simulink model "l64_dev"  (Simulink 7.9)
settings: Solver=ode45  StartTime=0.0  StopTime=525000  RelTol=1e-3
undefined symbols (not defined in the file): sfp
libraries: xbsIndex_r4 x835, xps_library x23, casper_library_delays x22, casper_library_misc x3
(part 1 of 8)
settings Model: Creator=jkocz  LastModifiedBy=jkocz
settings DebuggingCC: FcnCallInpInsideContextMsg=Use local settings  StrictBusMsg=Warning
settings GRTTargetCC: CombineOutputUpdateFcns=off  GRTInterface=on

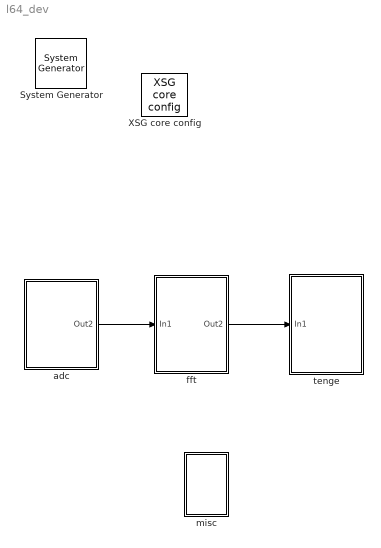
== system l64_dev ==
  " System Generator" : xbsIndex_r4/ System Generator  Tag=genX  xilinxfamily=virtex6  part=xc6vsx475t  speed=-1  package=ff1759  synthesis_tool=XST  clock_wrapper=Clock Enables  directory=./l64_dev/sysgen  proj_type=Project Navigator  Synth_file=XST Defaults  Impl_file=ISE Defaults  testbench=off  simulink_period=1  sysclk_period=5  dcm_input_clock_period=100  incr_netlist=off  trim_vbits=Everywhere in SubSystem  dbl_ovrd=According to Block Masks  core_generation=According to Block Masks  run_coregen=off  deprecated_control=off  eval_field=0  block_type=sysgen
      settings: block_version=11.4
  XSG core config : xps_library/XSG core config  Tag=xps:xsg  hw_sys=ROACH2:sx475t  clk_src=adc0_clk  ROACH_clk_src=adc0_clk  ROACH2_clk_src=adc0_clk  clk_rate=200  sample_period=1  synthesis_tool=XST
  adc : Subsystem
  fft : Subsystem
  misc : Subsystem
  tenge : Subsystem
  wires:
  adc/1(Out2) -> fft/1(In1)
  fft/1(Out2) -> tenge/1(In1)

== system l64_dev/adc ==
  Constant2 : Constant  Value=0
  Constant3 : Constant  Value=0
  Mux : Mux  Inputs=2
  Out2 : Outport
  wires:
  Mux/1 -> Out2/1
  Constant2/1 -> Mux/1
  Constant3/1 -> Mux/2

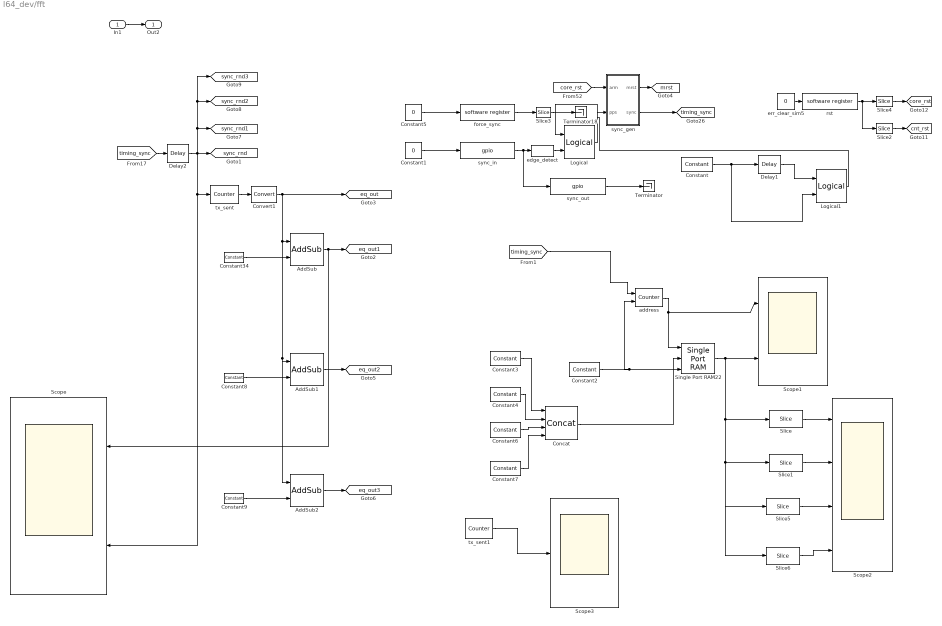
== system l64_dev/fft ==
  In1 : Inport
  AddSub : xbsIndex_r4/AddSub  mode=Addition  use_carryin=off  use_carryout=off  en=off  latency=0  precision=User Defined  arith_type=Unsigned  n_bits=64  bin_pt=0  quantization=Truncate  overflow=Wrap  dbl_ovrd=off  use_behavioral_HDL=off  hw_selection=Fabric  pipelined=off  block_type=addsub
  AddSub1 : xbsIndex_r4/AddSub  mode=Addition  use_carryin=off  use_carryout=off  en=off  latency=0  precision=User Defined  arith_type=Unsigned  n_bits=64  bin_pt=0  quantization=Truncate  overflow=Wrap  dbl_ovrd=off  use_behavioral_HDL=off  hw_selection=Fabric  pipelined=off  block_type=addsub
  AddSub2 : xbsIndex_r4/AddSub  mode=Addition  use_carryin=off  use_carryout=off  en=off  latency=0  precision=User Defined  arith_type=Unsigned  n_bits=64  bin_pt=0  quantization=Truncate  overflow=Wrap  dbl_ovrd=off  use_behavioral_HDL=off  hw_selection=Fabric  pipelined=off  block_type=addsub
  Concat : xbsIndex_r4/Concat  num_inputs=4  dbl_ovrd=off  block_type=concat
  Constant : xbsIndex_r4/Constant  const=1  gui_display_data_type=Boolean  arith_type=Boolean  n_bits=16  bin_pt=14  preci_type=Single  exp_width=8  frac_width=24  explicit_period=on  period=1  equ=P=C  opselect=C  inp2=PCIN>>17  opr=+  inp1=P  carry=CIN  dbl_ovrd=off  block_type=constant
  Constant1 : Constant  Value=0  SampleTime=1/4
  Constant2 : xbsIndex_r4/Constant  const=1  gui_display_data_type=Boolean  arith_type=Boolean  n_bits=16  bin_pt=14  preci_type=Single  exp_width=8  frac_width=24  explicit_period=on  period=1  equ=P=C  opselect=C  inp2=PCIN>>17  opr=+  inp1=P  carry=CIN  dbl_ovrd=off  block_type=constant
  Constant{3..4,6..7} (4 alike) : xbsIndex_r4/Constant  const=65536  gui_display_data_type=Fixed-point  arith_type=Unsigned  n_bits=16  bin_pt=0  preci_type=Single  exp_width=8  frac_width=24  explicit_period=on  period=1  equ=P=C  opselect=C  inp2=PCIN>>17  opr=+  inp1=P  carry=CIN  dbl_ovrd=off  block_type=constant
  Constant34 : xbsIndex_r4/Constant  const=8192  gui_display_data_type=Fixed-point  arith_type=Unsigned  n_bits=14  bin_pt=0  preci_type=Single  exp_width=8  frac_width=24  explicit_period=on  period=1  equ=P=C  opselect=C  inp2=PCIN>>17  opr=+  inp1=P  carry=CIN  dbl_ovrd=off  block_type=constant
  Constant5 : Constant  Value=0  SampleTime=1/4
  Constant8 : xbsIndex_r4/Constant  const=16384  gui_display_data_type=Fixed-point  arith_type=Unsigned  n_bits=15  bin_pt=0  preci_type=Single  exp_width=8  frac_width=24  explicit_period=on  period=1  equ=P=C  opselect=C  inp2=PCIN>>17  opr=+  inp1=P  carry=CIN  dbl_ovrd=off  block_type=constant
  Constant9 : xbsIndex_r4/Constant  const=24576  gui_display_data_type=Fixed-point  arith_type=Unsigned  n_bits=16  bin_pt=0  preci_type=Single  exp_width=8  frac_width=24  explicit_period=on  period=1  equ=P=C  opselect=C  inp2=PCIN>>17  opr=+  inp1=P  carry=CIN  dbl_ovrd=off  block_type=constant
  Convert1 : xbsIndex_r4/Convert  gui_display_data_type=Fixed-point  arith_type=Unsigned  n_bits=64  bin_pt=0  float_type=Single  exp_bits=8  fraction_bits=24  quantization=Truncate  overflow=Wrap  en=off  latency=0  dbl_ovrd=off  pipeline=off  block_type=convert
      settings: block_version=11.4
  Delay1 : xbsIndex_r4/Delay  rst=off  infoeditControl=Selection of Reset will increase slice count due to use of real FFs and instead of SRLs  en=off  latency=2  dbl_ovrd=off  reg_retiming=on  block_type=delay
  Delay2 : xbsIndex_r4/Delay  rst=off  infoeditControl=Selection of Reset will increase slice count due to use of real FFs and instead of SRLs  en=off  latency=10  dbl_ovrd=off  reg_retiming=on  block_type=delay
  Logical : xbsIndex_r4/Logical  logical_function=OR  inputs=2  en=off  latency=0  precision=Full  arith_type=Unsigned  n_bits=16  bin_pt=0  align_bp=on  dbl_ovrd=off  block_type=logical
  Logical1 : xbsIndex_r4/Logical  logical_function=OR  inputs=2  en=off  latency=0  precision=Full  arith_type=Unsigned  n_bits=16  bin_pt=0  align_bp=on  dbl_ovrd=off  block_type=logical
  Scope : Scope  NumInputPorts=2
      settings: YMin=0~-1  YMax=2e+19~1
  Scope1 : Scope  NumInputPorts=2
      settings: YMin=0~0  YMax=200~8500
  Scope2 : Scope  NumInputPorts=4
      settings: YMin=0~0~-5~-5  YMax=200~8500~5~5  SaveName=ScopeData2
  Scope3 : Scope
      settings: YMin=0  YMax=200  SaveName=ScopeData6
  Single Port RAM22 : xbsIndex_r4/Single Port RAM  depth=200  initVector=0  distributed_mem=Block RAM  write_mode=Read Before Write  rst=off  init_reg=0  en=off  latency=1  dbl_ovrd=off  optimize=Area  use_rpm=on  block_type=spram
  Slice : xbsIndex_r4/Slice  nbits=16  boolean_output=off  mode=Upper Bit Location + Width  bit1=0  base1=MSB of Input  bit0=0  base0=LSB of Input  dbl_ovrd=off  block_type=slice
  Slice1 : xbsIndex_r4/Slice  nbits=16  boolean_output=off  mode=Lower Bit Location + Width  bit1=0  base1=MSB of Input  bit0=32  base0=LSB of Input  dbl_ovrd=off  block_type=slice
  Slice2 : xbsIndex_r4/Slice  nbits=1  boolean_output=on  mode=Lower Bit Location + Width  bit1=0  base1=MSB of Input  bit0=0  base0=LSB of Input  dbl_ovrd=off  block_type=slice
      settings: block_version=10.1.3
  Slice3 : xbsIndex_r4/Slice  nbits=1  boolean_output=on  mode=Lower Bit Location + Width  bit1=0  base1=MSB of Input  bit0=0  base0=LSB of Input  dbl_ovrd=off  block_type=slice
      settings: block_version=10.1.3
  Slice4 : xbsIndex_r4/Slice  nbits=1  boolean_output=on  mode=Lower Bit Location + Width  bit1=0  base1=MSB of Input  bit0=1  base0=LSB of Input  dbl_ovrd=off  block_type=slice
      settings: block_version=10.1.3
  Slice5 : xbsIndex_r4/Slice  nbits=16  boolean_output=off  mode=Lower Bit Location + Width  bit1=0  base1=MSB of Input  bit0=16  base0=LSB of Input  dbl_ovrd=off  block_type=slice
  Slice6 : xbsIndex_r4/Slice  nbits=16  boolean_output=off  mode=Lower Bit Location + Width  bit1=0  base1=MSB of Input  bit0=0  base0=LSB of Input  dbl_ovrd=off  block_type=slice
  Terminator : Terminator
  Terminator18 : Terminator
  address : xbsIndex_r4/Counter  cnt_type=Count Limited  cnt_to=199  operation=Up  start_count=0  cnt_by_val=1  arith_type=Unsigned  n_bits=8  bin_pt=0  load_pin=off  rst=on  en=on  explicit_period=on  period=1  dbl_ovrd=off  use_behavioral_HDL=off  implementation=Fabric  block_type=counter
      settings: block_version=11.4
  edge_detect : casper_library_misc/edge_detect  edge=Rising  polarity=Active High  x_in=[0 0.08 0.08 0.16 0.16 0.24 0.24 0.32 0.32 0.4]  y_in="[-1 -1  1  1  1  1  1  1  1  1]"  x_out=[0.6 0.68 0.68 0.76 0.76 0.84 0.84 0.92 0.92 1]  y_out="[-1 -1  1  1 -1 -1 -1 -1 -1 -1]"
  err_clear_sim5 : Constant  Value=0
  force_sync : xps_library/software register  Tag=xps:sw_reg  io_dir=From Processor  arith_type=Unsigned  bitwidth=32  bin_pt=0  sample_period=1  gw_name=l64_dev_fft_force_sync_user_data_out
      link override r_10gbe_demo_gbe_core_rst_user_data_out: arith_type=Unsigned  n_bits=32  bin_pt=0  period=1
      link override r_10gbe_test_cnt_rst_user_data_out: arith_type=Unsigned  n_bits=32  bin_pt=0  period=1
      link override r_10gbe_test_gbe_core_rst_user_data_out: arith_type=Unsigned  n_bits=32  bin_pt=0  period=1
      link override r_xaui_test_cnt_rst_user_data_out: arith_type=Unsigned  n_bits=32  bin_pt=0  period=1
  rst : xps_library/software register  Tag=xps:sw_reg  io_dir=From Processor  arith_type=Unsigned  bitwidth=32  bin_pt=0  sample_period=1  gw_name=l64_dev_fft_rst_user_data_out
      link override r_10gbe_demo_gbe_core_rst_user_data_out: arith_type=Unsigned  n_bits=32  bin_pt=0  period=1
      link override r_10gbe_test_cnt_rst_user_data_out: arith_type=Unsigned  n_bits=32  bin_pt=0  period=1
      link override r_10gbe_test_gbe_core_rst_user_data_out: arith_type=Unsigned  n_bits=32  bin_pt=0  period=1
      link override r_xaui_test_cnt_rst_user_data_out: arith_type=Unsigned  n_bits=32  bin_pt=0  period=1
  sync_gen : Subsystem  mask(sync_gen_hw){sync_period_bits=14}
      mask prompts: sync_period_bits "Size of sync generator counter (bits)"
      mask help:
      | This circuit implements a scheme for synchronizing a design to within an FPGA clock of an external 1 pulse-per-second signal.
      |
      | * An arm pulse will cause the sync_gen to stop issuing sync pulses.
      | * It will then ignore the next input trigger (1PPS), while sync is flushed through the DSP pipeline.
      | * It will then lock onto the next trigger (1PPS) and issue syncs thereafter every sync_period clocks.
      | * You will need a multiple of (pfb_fir taps*LCM(FFT reorder orders) *fft bins/parallel inputs). See the sync memo for further details.
  sync_in : xps_library/gpio  Tag=xps:gpio  io_group=ROACH2:sync_in  io_dir=in  arith_type=Boolean  bitwidth=1  bin_pt=0  bit_index=0  sample_period=1  use_single_ended=off  use_ddr=off  reg_iob=on  reg_clk_phase=0  termination=None
  sync_out : xps_library/gpio  Tag=xps:gpio  io_group=ROACH2:sync_out  io_dir=out  arith_type=Boolean  bitwidth=1  bin_pt=0  bit_index=0  sample_period=1  use_single_ended=off  use_ddr=off  reg_iob=on  reg_clk_phase=0  termination=None
  tx_sent : xbsIndex_r4/Counter  cnt_type=Free Running  cnt_to=Inf  operation=Up  start_count=0  cnt_by_val=1  arith_type=Unsigned  n_bits=13  bin_pt=0  load_pin=off  rst=on  en=off  explicit_period=on  period=1  dbl_ovrd=off  use_behavioral_HDL=off  implementation=Fabric  block_type=counter
      settings: block_version=11.4
  tx_sent1 : xbsIndex_r4/Counter  cnt_type=Count Limited  cnt_to=10  operation=Up  start_count=0  cnt_by_val=1  arith_type=Unsigned  n_bits=13  bin_pt=0  load_pin=off  rst=off  en=off  explicit_period=on  period=1  dbl_ovrd=off  use_behavioral_HDL=off  implementation=Fabric  block_type=counter
      settings: block_version=11.4
  Out2 : Outport
  tag scope: cnt_rst=global, core_rst=global, eq_out1=global, eq_out2=global, eq_out3=global, eq_out=global, mrst=global, sync_rnd1=global, sync_rnd2=global, sync_rnd3=global, sync_rnd=global, timing_sync=global
  wires:
  In1/1 -> Out2/1
  [timing_sync] -> Delay2/1
  tx_sent/1 -> Convert1/1
  sync_gen/1(mrst) -> [mrst]
  sync_gen/2(sync) -> [timing_sync]
  [core_rst] -> sync_gen/1(arm)
  err_clear_sim5/1 -> rst/1
  rst/1 -> Slice4/1, Slice2/1
  Slice2/1 -> [cnt_rst]
  Slice4/1 -> [core_rst]
  force_sync/1 -> Slice3/1
  Constant5/1 -> force_sync/1
  Constant1/1 -> sync_in/1
  Logical/1 -> sync_gen/2(pps)
  sync_in/1 -> sync_out/1, edge_detect/1
  sync_out/1 -> Terminator/1
  edge_detect/1 -> Logical/2
  Slice3/1 -> Terminator18/1
  Constant/1 -> Delay1/1, Logical1/2
  Delay1/1 -> Logical1/1
  Logical1/1 -> Logical/1
  Delay2/1 -> [sync_rnd], tx_sent/1, Scope/2, [sync_rnd3], [sync_rnd2], [sync_rnd1]
  Constant2/1 -> Single Port RAM22/3, address/2
  Single Port RAM22/1 -> Scope1/2, Slice/1, Slice1/1, Slice5/1, Slice6/1
  address/1 -> Single Port RAM22/1, Scope1/1
  [timing_sync] -> address/1
  Convert1/1 -> [eq_out], AddSub/1, AddSub1/1, AddSub2/1
  Constant3/1 -> Concat/1
  Constant4/1 -> Concat/2
  Constant6/1 -> Concat/3
  Constant7/1 -> Concat/4
  Concat/1 -> Single Port RAM22/2
  Slice/1 -> Scope2/1
  Slice1/1 -> Scope2/2
  Slice5/1 -> Scope2/3
  Slice6/1 -> Scope2/4
  Constant34/1 -> AddSub/2
  AddSub/1 -> [eq_out1], Scope/1
  Constant8/1 -> AddSub1/2
  AddSub1/1 -> [eq_out2]
  Constant9/1 -> AddSub2/2
  AddSub2/1 -> [eq_out3]
  tx_sent1/1 -> Scope3/1

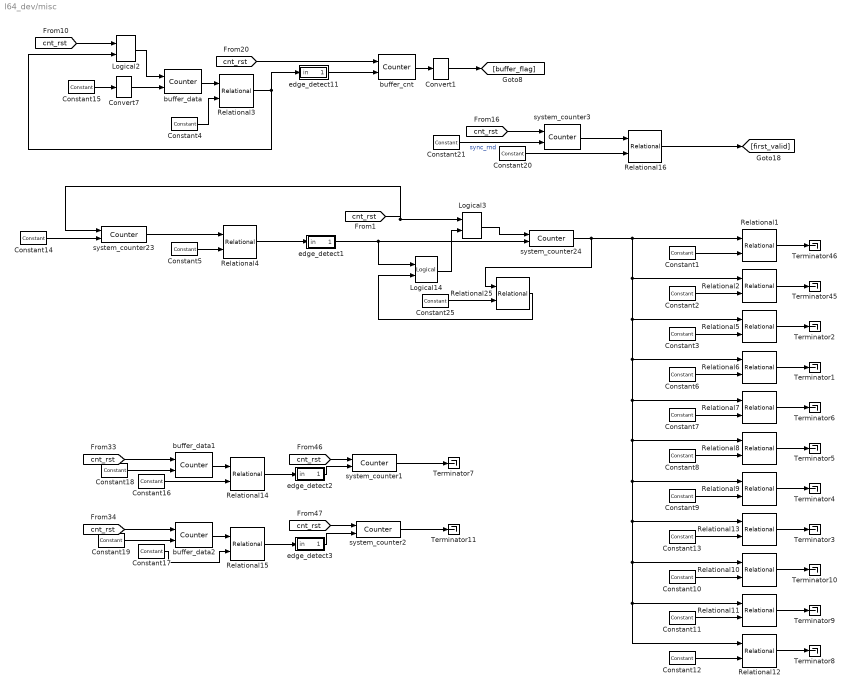
== system l64_dev/misc ==
  Constant1 : xbsIndex_r4/Constant  const=0  gui_display_data_type=Fixed-point  arith_type=Unsigned  n_bits=3  bin_pt=0  preci_type=Single  exp_width=8  frac_width=24  explicit_period=on  period=1  equ=P=C  opselect=C  inp2=PCIN>>17  opr=+  inp1=P  carry=CIN  dbl_ovrd=off  block_type=constant
  Constant10 : xbsIndex_r4/Constant  const=8  gui_display_data_type=Fixed-point  arith_type=Unsigned  n_bits=4  bin_pt=0  preci_type=Single  exp_width=8  frac_width=24  explicit_period=on  period=1  equ=P=C  opselect=C  inp2=PCIN>>17  opr=+  inp1=P  carry=CIN  dbl_ovrd=off  block_type=constant
  Constant11 : xbsIndex_r4/Constant  const=9  gui_display_data_type=Fixed-point  arith_type=Unsigned  n_bits=4  bin_pt=0  preci_type=Single  exp_width=8  frac_width=24  explicit_period=on  period=1  equ=P=C  opselect=C  inp2=PCIN>>17  opr=+  inp1=P  carry=CIN  dbl_ovrd=off  block_type=constant
  Constant{12,16..17,25} (4 alike) : xbsIndex_r4/Constant  const=10  gui_display_data_type=Fixed-point  arith_type=Unsigned  n_bits=4  bin_pt=0  preci_type=Single  exp_width=8  frac_width=24  explicit_period=on  period=1  equ=P=C  opselect=C  inp2=PCIN>>17  opr=+  inp1=P  carry=CIN  dbl_ovrd=off  block_type=constant
  Constant13 : xbsIndex_r4/Constant  const=7  gui_display_data_type=Fixed-point  arith_type=Unsigned  n_bits=3  bin_pt=0  preci_type=Single  exp_width=8  frac_width=24  explicit_period=on  period=1  equ=P=C  opselect=C  inp2=PCIN>>17  opr=+  inp1=P  carry=CIN  dbl_ovrd=off  block_type=constant
  Constant{14..15,18..19,21} (5 alike) : xbsIndex_r4/Constant  const=0  gui_display_data_type=Boolean  arith_type=Boolean  n_bits=9  bin_pt=0  preci_type=Single  exp_width=8  frac_width=24  explicit_period=on  period=1  equ=P=C  opselect=C  inp2=PCIN>>17  opr=+  inp1=P  carry=CIN  dbl_ovrd=off  block_type=constant
  Constant2 : xbsIndex_r4/Constant  const=1  gui_display_data_type=Fixed-point  arith_type=Unsigned  n_bits=3  bin_pt=0  preci_type=Single  exp_width=8  frac_width=24  explicit_period=on  period=1  equ=P=C  opselect=C  inp2=PCIN>>17  opr=+  inp1=P  carry=CIN  dbl_ovrd=off  block_type=constant
  Constant20 : xbsIndex_r4/Constant  const=1  gui_display_data_type=Fixed-point  arith_type=Unsigned  n_bits=2  bin_pt=0  preci_type=Single  exp_width=8  frac_width=24  explicit_period=on  period=1  equ=P=C  opselect=C  inp2=PCIN>>17  opr=+  inp1=P  carry=CIN  dbl_ovrd=off  block_type=constant
  Constant3 : xbsIndex_r4/Constant  const=2  gui_display_data_type=Fixed-point  arith_type=Unsigned  n_bits=3  bin_pt=0  preci_type=Single  exp_width=8  frac_width=24  explicit_period=on  period=1  equ=P=C  opselect=C  inp2=PCIN>>17  opr=+  inp1=P  carry=CIN  dbl_ovrd=off  block_type=constant
  Constant4 : xbsIndex_r4/Constant  const=22  gui_display_data_type=Fixed-point  arith_type=Unsigned  n_bits=5  bin_pt=0  preci_type=Single  exp_width=8  frac_width=24  explicit_period=on  period=1  equ=P=C  opselect=C  inp2=PCIN>>17  opr=+  inp1=P  carry=CIN  dbl_ovrd=off  block_type=constant
  Constant5 : xbsIndex_r4/Constant  const=109  gui_display_data_type=Fixed-point  arith_type=Unsigned  n_bits=9  bin_pt=0  preci_type=Single  exp_width=8  frac_width=24  explicit_period=on  period=1  equ=P=C  opselect=C  inp2=PCIN>>17  opr=+  inp1=P  carry=CIN  dbl_ovrd=off  block_type=constant
  Constant6 : xbsIndex_r4/Constant  const=3  gui_display_data_type=Fixed-point  arith_type=Unsigned  n_bits=3  bin_pt=0  preci_type=Single  exp_width=8  frac_width=24  explicit_period=on  period=1  equ=P=C  opselect=C  inp2=PCIN>>17  opr=+  inp1=P  carry=CIN  dbl_ovrd=off  block_type=constant
  Constant7 : xbsIndex_r4/Constant  const=4  gui_display_data_type=Fixed-point  arith_type=Unsigned  n_bits=3  bin_pt=0  preci_type=Single  exp_width=8  frac_width=24  explicit_period=on  period=1  equ=P=C  opselect=C  inp2=PCIN>>17  opr=+  inp1=P  carry=CIN  dbl_ovrd=off  block_type=constant
  Constant8 : xbsIndex_r4/Constant  const=5  gui_display_data_type=Fixed-point  arith_type=Unsigned  n_bits=3  bin_pt=0  preci_type=Single  exp_width=8  frac_width=24  explicit_period=on  period=1  equ=P=C  opselect=C  inp2=PCIN>>17  opr=+  inp1=P  carry=CIN  dbl_ovrd=off  block_type=constant
  Constant9 : xbsIndex_r4/Constant  const=6  gui_display_data_type=Fixed-point  arith_type=Unsigned  n_bits=3  bin_pt=0  preci_type=Single  exp_width=8  frac_width=24  explicit_period=on  period=1  equ=P=C  opselect=C  inp2=PCIN>>17  opr=+  inp1=P  carry=CIN  dbl_ovrd=off  block_type=constant
  Convert1 : xbsIndex_r4/Convert  gui_display_data_type=Boolean  arith_type=Boolean  n_bits=64  bin_pt=0  float_type=Single  exp_bits=8  fraction_bits=24  quantization=Truncate  overflow=Wrap  en=off  latency=0  dbl_ovrd=off  pipeline=off  block_type=convert
      settings: block_version=11.4
  Convert7 : xbsIndex_r4/Convert  gui_display_data_type=Boolean  arith_type=Boolean  n_bits=64  bin_pt=0  float_type=Single  exp_bits=8  fraction_bits=24  quantization=Truncate  overflow=Wrap  en=off  latency=0  dbl_ovrd=off  pipeline=off  block_type=convert
      settings: block_version=11.4
  Logical14 : xbsIndex_r4/Logical  logical_function=AND  inputs=2  en=off  latency=0  precision=Full  arith_type=Unsigned  n_bits=16  bin_pt=0  align_bp=on  dbl_ovrd=off  block_type=logical
      settings: block_version=11.4
  Logical2 : xbsIndex_r4/Logical  logical_function=OR  inputs=2  en=off  latency=1  precision=Full  arith_type=Unsigned  n_bits=16  bin_pt=0  align_bp=on  dbl_ovrd=off  block_type=logical
      settings: block_version=11.4
  Logical3 : xbsIndex_r4/Logical  logical_function=OR  inputs=2  en=off  latency=1  precision=Full  arith_type=Unsigned  n_bits=16  bin_pt=0  align_bp=on  dbl_ovrd=off  block_type=logical
      settings: block_version=11.4
  Relational{1..15,25} (16 alike) : xbsIndex_r4/Relational  mode=a=b  en=off  latency=0  dbl_ovrd=off  block_type=relational
      settings: xl_area=[0, 0, 0, 0, 0, 0, 0]  block_version=10.1.3
  Relational16 : xbsIndex_r4/Relational  mode=a>=b  en=off  latency=0  dbl_ovrd=off  block_type=relational
      settings: xl_area=[0, 0, 0, 0, 0, 0, 0]  block_version=10.1.3
  Terminator{1..11,45..46} (13 alike) : Terminator
  buffer_cnt : xbsIndex_r4/Counter  cnt_type=Free Running  cnt_to=Inf  operation=Up  start_count=0  cnt_by_val=1  arith_type=Unsigned  n_bits=1  bin_pt=0  load_pin=off  rst=on  en=on  explicit_period=on  period=1  dbl_ovrd=off  use_behavioral_HDL=off  implementation=Fabric  block_type=counter
      settings: block_version=11.4
  buffer_data : xbsIndex_r4/Counter  cnt_type=Free Running  cnt_to=Inf  operation=Up  start_count=0  cnt_by_val=1  arith_type=Unsigned  n_bits=5  bin_pt=0  load_pin=off  rst=on  en=on  explicit_period=on  period=1  dbl_ovrd=off  use_behavioral_HDL=off  implementation=Fabric  block_type=counter
      settings: block_version=11.4
  buffer_data1 : xbsIndex_r4/Counter  cnt_type=Count Limited  cnt_to=10  operation=Up  start_count=0  cnt_by_val=1  arith_type=Unsigned  n_bits=4  bin_pt=0  load_pin=off  rst=on  en=on  explicit_period=on  period=1  dbl_ovrd=off  use_behavioral_HDL=off  implementation=Fabric  block_type=counter
      settings: block_version=11.4
  buffer_data2 : xbsIndex_r4/Counter  cnt_type=Count Limited  cnt_to=10  operation=Up  start_count=0  cnt_by_val=1  arith_type=Unsigned  n_bits=4  bin_pt=0  load_pin=off  rst=on  en=on  explicit_period=on  period=1  dbl_ovrd=off  use_behavioral_HDL=off  implementation=Fabric  block_type=counter
      settings: block_version=11.4
  edge_detect1 : Subsystem  AncestorBlock=casper_library_misc/edge_detect  mask(edge_detect){edge=Rising, polarity=Active High, x_in=[0 0.08 0.08 0.16 0.16 0.24 0.24 0.32 0.32 0.4], y_in=[-1 -1  1  1  1  1  1  1  1  1], x_out=[0.6 0.68 0.68 0.76 0.76 0.84 0.84 0.92 0.92 1], y_out=[-1 -1  1  1 -1 -1 -1 -1 -1 -1]}
      mask prompts: edge "Edge Type"; polarity "Output Polarity"; x_in "Input X Positions"; y_in "Input Y Positions"; x_out "Output X Positions"; y_out "Output Y Positions"
      mask help: Output is active for one-cycle after each edge of the specified type (i.e. rising, falling or both).
      mask init:
      | edge_detect_init(gcb,...
      |     'edge',edge,...
      |     'polarity',polarity,...
      |     'x_in',x_in,...
      |     'x_out',x_out,...
      |     'y_in',y_in,...
      |     'y_out',y_out);
      | 
      | x_in_num=str2num(getfield(getfield(get_param(gcb,'UserData'),'parameters'),'x_in'));
      | x_out_num=str2num(getfield(getfield(get_param(gcb,'UserData'),'parameters'),'x_out'));
      | y_in_num=str2num(getfield(getfield(get_param(gcb,'UserData'),'parameters'),'y_in'));
      | y_out_num=str2num(getfield(getfield(get_param(gcb,'UserData'),'parameters'),'y_out'));
      settings: AttributesFormatString=|
      | rising edges
      | active high
      mask Help: Output is active for one-cycle after each edge of the specified type (i.e. rising, falling, or both).  Latency is zero.
      mask StyleString: popup(Rising|Falling|Both),popup(Active High|Active Low),edit,edit,edit,edit
      mask Display:
      | plot(x_in_num,0.5+y_in_num*0.2);
      | plot(x_out_num,0.5+y_out_num*0.2);
  edge_detect11 : Subsystem  AncestorBlock=casper_library_misc/edge_detect  mask(edge_detect){edge=Rising, polarity=Active High, x_in=[0 0.08 0.08 0.16 0.16 0.24 0.24 0.32 0.32 0.4], y_in=[-1 -1  1  1  1  1  1  1  1  1], x_out=[0.6 0.68 0.68 0.76 0.76 0.84 0.84 0.92 0.92 1], y_out=[-1 -1  1  1 -1 -1 -1 -1 -1 -1]}
      mask prompts: edge "Edge Type"; polarity "Output Polarity"; x_in "Input X Positions"; y_in "Input Y Positions"; x_out "Output X Positions"; y_out "Output Y Positions"
      mask help: Output is active for one-cycle after each edge of the specified type (i.e. rising, falling or both).
      mask init: same as l64_dev/misc/edge_detect1
      settings: AttributesFormatString=|
      | rising edges
      | active high
      mask Help: Output is active for one-cycle after each edge of the specified type (i.e. rising, falling, or both).  Latency is zero.
      mask StyleString: popup(Rising|Falling|Both),popup(Active High|Active Low),edit,edit,edit,edit
      mask Display:
      | plot(x_in_num,0.5+y_in_num*0.2);
      | plot(x_out_num,0.5+y_out_num*0.2);
  edge_detect2 : Subsystem  AncestorBlock=casper_library_misc/edge_detect  mask(edge_detect){edge=Rising, polarity=Active High, x_in=[0 0.08 0.08 0.16 0.16 0.24 0.24 0.32 0.32 0.4], y_in=[-1 -1  1  1  1  1  1  1  1  1], x_out=[0.6 0.68 0.68 0.76 0.76 0.84 0.84 0.92 0.92 1], y_out=[-1 -1  1  1 -1 -1 -1 -1 -1 -1]}
      mask prompts: edge "Edge Type"; polarity "Output Polarity"; x_in "Input X Positions"; y_in "Input Y Positions"; x_out "Output X Positions"; y_out "Output Y Positions"
      mask help: Output is active for one-cycle after each edge of the specified type (i.e. rising, falling or both).
      mask init: same as l64_dev/misc/edge_detect1
      settings: AttributesFormatString=|
      | rising edges
      | active high
      mask Help: Output is active for one-cycle after each edge of the specified type (i.e. rising, falling, or both).  Latency is zero.
      mask StyleString: popup(Rising|Falling|Both),popup(Active High|Active Low),edit,edit,edit,edit
      mask Display:
      | plot(x_in_num,0.5+y_in_num*0.2);
      | plot(x_out_num,0.5+y_out_num*0.2);
  edge_detect3 : Subsystem  AncestorBlock=casper_library_misc/edge_detect  mask(edge_detect){edge=Rising, polarity=Active High, x_in=[0 0.08 0.08 0.16 0.16 0.24 0.24 0.32 0.32 0.4], y_in=[-1 -1  1  1  1  1  1  1  1  1], x_out=[0.6 0.68 0.68 0.76 0.76 0.84 0.84 0.92 0.92 1], y_out=[-1 -1  1  1 -1 -1 -1 -1 -1 -1]}
      mask prompts: edge "Edge Type"; polarity "Output Polarity"; x_in "Input X Positions"; y_in "Input Y Positions"; x_out "Output X Positions"; y_out "Output Y Positions"
      mask help: Output is active for one-cycle after each edge of the specified type (i.e. rising, falling or both).
      mask init: same as l64_dev/misc/edge_detect1
      settings: AttributesFormatString=|
      | rising edges
      | active high
      mask Help: Output is active for one-cycle after each edge of the specified type (i.e. rising, falling, or both).  Latency is zero.
      mask StyleString: popup(Rising|Falling|Both),popup(Active High|Active Low),edit,edit,edit,edit
      mask Display:
      | plot(x_in_num,0.5+y_in_num*0.2);
      | plot(x_out_num,0.5+y_out_num*0.2);
  system_counter1 : xbsIndex_r4/Counter  cnt_type=Count Limited  cnt_to=10  operation=Up  start_count=0  cnt_by_val=1  arith_type=Unsigned  n_bits=4  bin_pt=0  load_pin=off  rst=on  en=on  explicit_period=on  period=1  dbl_ovrd=off  use_behavioral_HDL=off  implementation=Fabric  block_type=counter
      settings: block_version=11.4
  system_counter2 : xbsIndex_r4/Counter  cnt_type=Count Limited  cnt_to=10  operation=Up  start_count=0  cnt_by_val=1  arith_type=Unsigned  n_bits=4  bin_pt=0  load_pin=off  rst=on  en=on  explicit_period=on  period=1  dbl_ovrd=off  use_behavioral_HDL=off  implementation=Fabric  block_type=counter
      settings: block_version=11.4
  system_counter23 : xbsIndex_r4/Counter  cnt_type=Count Limited  cnt_to=435  operation=Up  start_count=0  cnt_by_val=1  arith_type=Unsigned  n_bits=9  bin_pt=0  load_pin=off  rst=on  en=on  explicit_period=on  period=1  dbl_ovrd=off  use_behavioral_HDL=off  implementation=Fabric  block_type=counter
      settings: block_version=11.4
  system_counter24 : xbsIndex_r4/Counter  cnt_type=Count Limited  cnt_to=10  operation=Up  start_count=0  cnt_by_val=1  arith_type=Unsigned  n_bits=8  bin_pt=0  load_pin=off  rst=on  en=on  explicit_period=on  period=1  dbl_ovrd=off  use_behavioral_HDL=off  implementation=Fabric  block_type=counter
      settings: block_version=11.4
  system_counter3 : xbsIndex_r4/Counter  cnt_type=Free Running  cnt_to=Inf  operation=Up  start_count=0  cnt_by_val=1  arith_type=Unsigned  n_bits=64  bin_pt=0  load_pin=off  rst=on  en=on  explicit_period=on  period=1  dbl_ovrd=off  use_behavioral_HDL=off  implementation=Fabric  block_type=counter
      settings: block_version=11.4
  wires:
  buffer_cnt/1 -> Convert1/1
  [cnt_rst] -> buffer_cnt/1
  buffer_data/1 -> Relational3/1
  Constant4/1 -> Relational3/2
  Relational3/1 -> Logical2/2, edge_detect11/1(in)
  Constant15/1 -> Convert7/1
  [cnt_rst] -> Logical2/1
  Logical2/1 -> buffer_data/1
  edge_detect11/1(out) -> buffer_cnt/2
  Convert7/1 -> buffer_data/2
  Convert1/1 -> [buffer_flag]
  Constant14/1 -> system_counter23/2
  Constant5/1 -> Relational4/2
  edge_detect1/1(out) -> system_counter24/2, Logical14/1
  [cnt_rst] -> Logical3/1, system_counter23/1
  Relational4/1 -> edge_detect1/1(in)
  system_counter23/1 -> Relational4/1
  system_counter24/1 -> Relational1/1, Relational2/1, Relational5/1, Relational6/1, Relational7/1, Relational8/1, Relational9/1, Relational13/1, Relational10/1, Relational11/1, Relational12/1, Relational25/1
  Constant1/1 -> Relational1/2
  Relational1/1 -> Terminator46/1
  Constant2/1 -> Relational2/2
  Relational2/1 -> Terminator45/1
  Constant3/1 -> Relational5/2
  Constant6/1 -> Relational6/2
  Constant7/1 -> Relational7/2
  Constant8/1 -> Relational8/2
  Constant9/1 -> Relational9/2
  Constant13/1 -> Relational13/2
  Constant10/1 -> Relational10/2
  Constant11/1 -> Relational11/2
  Constant12/1 -> Relational12/2
  Logical3/1 -> system_counter24/1
  Constant25/1 -> Relational25/2
  Relational25/1 -> Logical14/2
  Logical14/1 -> Logical3/2
  Relational5/1 -> Terminator2/1
  Relational6/1 -> Terminator1/1
  Relational7/1 -> Terminator6/1
  Relational8/1 -> Terminator5/1
  Relational9/1 -> Terminator4/1
  Relational13/1 -> Terminator3/1
  Relational10/1 -> Terminator10/1
  Relational11/1 -> Terminator9/1
  Relational12/1 -> Terminator8/1
  buffer_data1/1 -> Relational14/1
  Constant16/1 -> Relational14/2
  Relational14/1 -> edge_detect2/1(in)
  Constant18/1 -> buffer_data1/2
  buffer_data2/1 -> Relational15/1
  Relational15/1 -> edge_detect3/1(in)
  Constant19/1 -> buffer_data2/2
  [cnt_rst] -> system_counter1/1
  [cnt_rst] -> system_counter2/1
  [cnt_rst] -> buffer_data1/1
  [cnt_rst] -> buffer_data2/1
  edge_detect2/1(out) -> system_counter1/2
  edge_detect3/1(out) -> system_counter2/2
  system_counter1/1 -> Terminator7/1
  system_counter2/1 -> Terminator11/1
  Constant17/1 -> Relational15/2
  system_counter3/1 -> Relational16/1
  Constant20/1 -> Relational16/2
  Relational16/1 -> [first_valid]
  [cnt_rst] -> system_counter3/1
  Constant21/1 -> system_counter3/2  "sync_rnd"

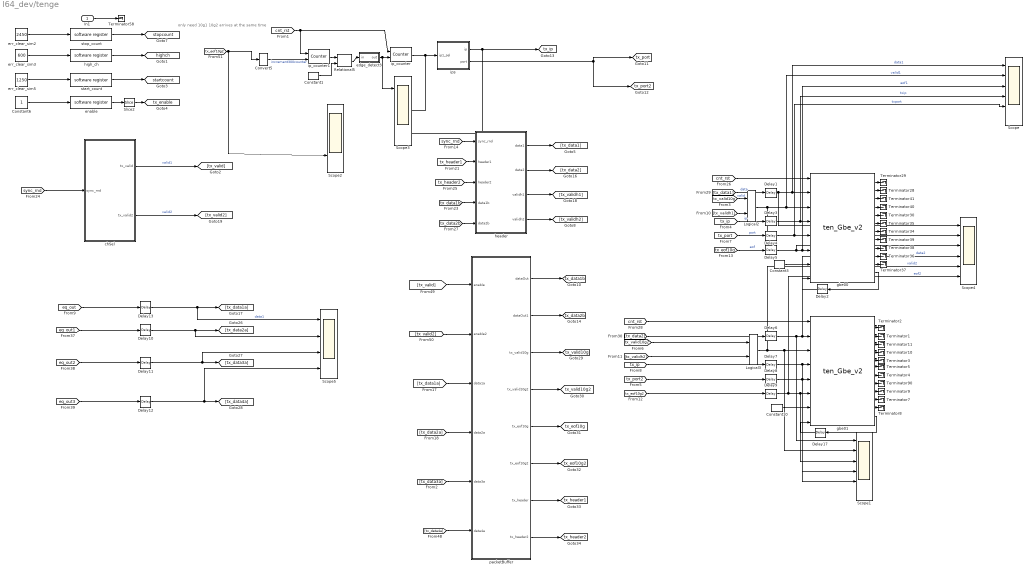
== system l64_dev/tenge ==
  note: only need 10g1
      | 10g2 arrives at the same time
  In1 : Inport
  Constant1 : xbsIndex_r4/Constant  const=1  gui_display_data_type=Fixed-point  arith_type=Unsigned  n_bits=2  bin_pt=0  preci_type=Single  exp_width=8  frac_width=24  explicit_period=on  period=1  equ=P=C  opselect=C  inp2=PCIN>>17  opr=+  inp1=P  carry=CIN  dbl_ovrd=off  block_type=constant
  Constant10 : xbsIndex_r4/Constant  const=1  gui_display_data_type=Fixed-point  arith_type=Boolean  n_bits=1  bin_pt=0  preci_type=Single  exp_width=8  frac_width=24  explicit_period=on  period=1  equ=P=C  opselect=C  inp2=PCIN>>17  opr=+  inp1=P  carry=CIN  dbl_ovrd=off  block_type=constant
  Constant3 : xbsIndex_r4/Constant  const=1  gui_display_data_type=Fixed-point  arith_type=Boolean  n_bits=1  bin_pt=0  preci_type=Single  exp_width=8  frac_width=24  explicit_period=on  period=1  equ=P=C  opselect=C  inp2=PCIN>>17  opr=+  inp1=P  carry=CIN  dbl_ovrd=off  block_type=constant
  Constant6 : Constant
  Convert5 : xbsIndex_r4/Convert  gui_display_data_type=Boolean  arith_type=Boolean  n_bits=64  bin_pt=0  float_type=Single  exp_bits=8  fraction_bits=24  quantization=Truncate  overflow=Wrap  en=off  latency=1  dbl_ovrd=off  pipeline=off  block_type=convert
      settings: block_version=11.4
  Delay{1..4,6..8,17} (8 alike) : xbsIndex_r4/Delay  rst=off  infoeditControl=Selection of Reset will increase slice count due to use of real FFs and instead of SRLs  en=off  latency=1  dbl_ovrd=off  reg_retiming=on  block_type=delay
  Delay{10..13} (4 alike) : xbsIndex_r4/Delay  rst=off  infoeditControl=Selection of Reset will increase slice count due to use of real FFs and instead of SRLs  en=off  latency=5  dbl_ovrd=off  reg_retiming=on  block_type=delay
      settings: xl_area=[0, 0, 0, 0, 0, 0, 0]
  Delay5 : xbsIndex_r4/Delay  rst=off  infoeditControl=Selection of Reset will increase slice count due to use of real FFs and instead of SRLs  en=off  latency=3  dbl_ovrd=off  reg_retiming=on  block_type=delay
  Delay9 : xbsIndex_r4/Delay  rst=off  infoeditControl=Selection of Reset will increase slice count due to use of real FFs and instead of SRLs  en=off  latency=3  dbl_ovrd=off  reg_retiming=on  block_type=delay
  Logical2 : xbsIndex_r4/Logical  logical_function=OR  inputs=2  en=off  latency=3  precision=Full  arith_type=Unsigned  n_bits=16  bin_pt=0  align_bp=on  dbl_ovrd=off  block_type=logical
      settings: block_version=11.4
  Logical3 : xbsIndex_r4/Logical  logical_function=OR  inputs=2  en=off  latency=3  precision=Full  arith_type=Unsigned  n_bits=16  bin_pt=0  align_bp=on  dbl_ovrd=off  block_type=logical
      settings: block_version=11.4
  Relational5 : xbsIndex_r4/Relational  mode=a=b  en=off  latency=1  dbl_ovrd=off  block_type=relational
      settings: xl_area=[0, 0, 0, 0, 0, 0, 0]  block_version=10.1.3
  Scope : Scope  NumInputPorts=6
      settings: TimeRange=125000  YMin=0~0~0~4012~3800.95~-1  YMax=7000~1~1~4022~4201.05~1  SaveName=ScopeData8
  Scope1 : Scope  NumInputPorts=6
      settings: YMin=0~0~0~0~0~-5  YMax=900~1~1~3~30000~5  SaveName=ScopeData9
  Scope2 : Scope  NumInputPorts=2
      settings: YMin=0~0  YMax=7000~1  SaveName=ScopeData7
  Scope3 : Scope  NumInputPorts=3
      settings: YMin=0~0~-5  YMax=7000~1~5  SaveName=ScopeData10
  Scope4 : Scope  NumInputPorts=6
      settings: TimeRange=125000  YMin=0~0~0~4012~3800.95~-1  YMax=7000~1~1~4022~4201.05~1  SaveName=ScopeData11
  Scope5 : Scope  NumInputPorts=4
      settings: YMin=0~0~-5~-5  YMax=7000~1~5~5  SaveName=ScopeData13
  Slice2 : xbsIndex_r4/Slice  nbits=1  boolean_output=off  mode=Lower Bit Location + Width  bit1=1  base1=MSB of Input  bit0=0  base0=LSB of Input  dbl_ovrd=off  block_type=slice
      settings: block_version=10.1.3
  Terminator{1..5,7..11,28..30,34..41,58,90} (23 alike) : Terminator
  chSel : Subsystem
  edge_detect3 : Subsystem  AncestorBlock=casper_library_misc/edge_detect  mask(edge_detect){edge=Rising, polarity=Active High, x_in=[0 0.08 0.08 0.16 0.16 0.24 0.24 0.32 0.32 0.4], y_in=[-1 -1  1  1  1  1  1  1  1  1], x_out=[0.6 0.68 0.68 0.76 0.76 0.84 0.84 0.92 0.92 1], y_out=[-1 -1  1  1 -1 -1 -1 -1 -1 -1]}
      mask prompts: edge "Edge Type"; polarity "Output Polarity"; x_in "Input X Positions"; y_in "Input Y Positions"; x_out "Output X Positions"; y_out "Output Y Positions"
      mask help: Output is active for one-cycle after each edge of the specified type (i.e. rising, falling or both).
      mask init: same as l64_dev/misc/edge_detect1
      settings: AttributesFormatString=|
      | rising edges
      | active high
      mask Help: Output is active for one-cycle after each edge of the specified type (i.e. rising, falling, or both).  Latency is zero.
      mask StyleString: popup(Rising|Falling|Both),popup(Active High|Active Low),edit,edit,edit,edit
      mask Display:
      | plot(x_in_num,0.5+y_in_num*0.2);
      | plot(x_out_num,0.5+y_out_num*0.2);
  enable : xps_library/software register  Tag=xps:sw_reg  io_dir=From Processor  arith_type=Unsigned  bitwidth=32  bin_pt=0  sample_period=1  gw_name=l64_dev_tenge_enable_user_data_out
      link override r_10gbe_demo_pkt_sim_run_user_data_out: arith_type=Unsigned  n_bits=32  bin_pt=0  period=1
      link override r_10gbe_test_pkt_sim_run_user_data_out: arith_type=Unsigned  n_bits=32  bin_pt=0  period=1
      link override test_pkt_buffer_10_1_p_mux_up_run_user_data_out: arith_type=Unsigned  n_bits=32  bin_pt=0  period=1
  err_clear_sim2 : Constant  Value=2450
  err_clear_sim3 : Constant  Value=600
  err_clear_sim5 : Constant  Value=1250
  gbe00 : xps_library/ten_Gbe_v2  Tag=xps:tengbe_v2  flavour=sfp+  slot=0  port_r1=0  port_r2_cx4=0  port_r2_sfpp=0  rx_dist_ram=off  large_frames=on  show_param=on  pre_emph_r2=0.74  pre_emph=3  post_emph_r2=0.18  rxeqmix_r2=7  swing_r2=940  swing=800  fab_en=off  fab_mac=hex2dec('123456789100')  fab_ip=192*(2^24) + 168*(2^16) + 5*(2^8) + 14*(2^0)  fab_udp=10002  fab_gate=192*(2^24) + 168*(2^16) + 5*(2^8) + 0  cpu_rx_en=on  cpu_tx_en=on
  gbe01 : xps_library/ten_Gbe_v2  Tag=xps:tengbe_v2  flavour=sfp+  slot=0  port_r1=0  port_r2_cx4=0  port_r2_sfpp=1  rx_dist_ram=off  large_frames=on  show_param=on  pre_emph_r2=0.74  pre_emph=3  post_emph_r2=0.18  rxeqmix_r2=7  swing_r2=940  swing=800  fab_en=off  fab_mac=hex2dec('123456789105')  fab_ip=192*(2^24) + 168*(2^16) + 6*(2^8) + 15*(2^0)  fab_udp=10002  fab_gate=192*(2^24) + 168*(2^16) + 6*(2^8) + 0  cpu_rx_en=on  cpu_tx_en=on
  header : Subsystem
  high_ch : xps_library/software register  Tag=xps:sw_reg  io_dir=From Processor  arith_type=Unsigned  bitwidth=32  bin_pt=0  sample_period=1  gw_name=l64_dev_tenge_high_ch_user_data_out
      link override r_10gbe_demo_dest_ip_user_data_out: arith_type=Unsigned  n_bits=32  bin_pt=0  period=1
      link override r_10gbe_test_dest_ip_user_data_out: arith_type=Unsigned  n_bits=32  bin_pt=0  period=1
      link override r_xaui_test_cnt_rst_user_data_out: arith_type=Unsigned  n_bits=32  bin_pt=0  period=1
  ip_counter : xbsIndex_r4/Counter  cnt_type=Free Running  cnt_to=3  operation=Up  start_count=0  cnt_by_val=1  arith_type=Unsigned  n_bits=2  bin_pt=0  load_pin=off  rst=on  en=on  explicit_period=on  period=1  dbl_ovrd=off  use_behavioral_HDL=off  implementation=Fabric  block_type=counter
      settings: block_version=11.4
  ip_counter1 : xbsIndex_r4/Counter  cnt_type=Free Running  cnt_to=0  operation=Up  start_count=1  cnt_by_val=1  arith_type=Unsigned  n_bits=1  bin_pt=0  load_pin=off  rst=on  en=on  explicit_period=on  period=1  dbl_ovrd=off  use_behavioral_HDL=off  implementation=Fabric  block_type=counter
      settings: block_version=11.4
  ips : Subsystem
  packetBuffer : Subsystem
  start_count : xps_library/software register  Tag=xps:sw_reg  io_dir=From Processor  arith_type=Unsigned  bitwidth=32  bin_pt=0  sample_period=1  gw_name=l64_dev_tenge_start_count_user_data_out
      link override r_10gbe_demo_dest_ip_user_data_out: arith_type=Unsigned  n_bits=32  bin_pt=0  period=1
      link override r_10gbe_test_dest_ip_user_data_out: arith_type=Unsigned  n_bits=32  bin_pt=0  period=1
      link override r_xaui_test_cnt_rst_user_data_out: arith_type=Unsigned  n_bits=32  bin_pt=0  period=1
  stop_count : xps_library/software register  Tag=xps:sw_reg  io_dir=From Processor  arith_type=Unsigned  bitwidth=32  bin_pt=0  sample_period=1  gw_name=l64_dev_tenge_stop_count_user_data_out
      link override leda_64_sim_tenge_stop_count_user_data_out: arith_type=Unsigned  n_bits=32  bin_pt=0  period=1
      link override r_10gbe_demo_dest_ip_user_data_out: arith_type=Unsigned  n_bits=32  bin_pt=0  period=1
      link override r_10gbe_test_dest_ip_user_data_out: arith_type=Unsigned  n_bits=32  bin_pt=0  period=1
      link override r_xaui_test_cnt_rst_user_data_out: arith_type=Unsigned  n_bits=32  bin_pt=0  period=1
  tag scope: highch=global, startcount=global, stopcount=global, tx_data1b=global, tx_data2b=global, tx_enable=global, tx_eof10g2=global, tx_eof10g=global, tx_header1=global, tx_header2=global, tx_ip=global, tx_port2=global, tx_port=global, tx_valid10g2=global, tx_valid10g=global
  wires:
  In1/1 -> Terminator58/1
  err_clear_sim2/1 -> stop_count/1
  stop_count/1 -> [stopcount]
  err_clear_sim3/1 -> high_ch/1
  high_ch/1 -> [highch]
  err_clear_sim5/1 -> start_count/1
  start_count/1 -> [startcount]
  enable/1 -> Slice2/1
  Constant6/1 -> enable/1
  Slice2/1 -> [tx_enable]
  [sync_rnd] -> chSel/1(sync_rnd)
  gbe00/12 -> Delay2/1
  Delay2/1 -> gbe00/8
  gbe00/5 -> Terminator30/1
  gbe00/4 -> Terminator40/1
  gbe00/9 -> Terminator38/1
  gbe00/1 -> Terminator29/1
  gbe00/2 -> Terminator28/1
  gbe00/3 -> Terminator41/1
  gbe00/6 -> Terminator35/1
  gbe00/7 -> Terminator34/1
  gbe00/8 -> Terminator39/1
  gbe00/10 -> Terminator36/1
  gbe00/11 -> Terminator37/1
  [cnt_rst] -> gbe00/1
  Constant10/1 -> gbe01/7
  gbe01/12 -> Delay17/1
  Delay17/1 -> gbe01/8
  gbe01/5 -> Terminator3/1
  gbe01/4 -> Terminator10/1
  gbe01/9 -> Terminator9/1
  gbe01/1 -> Terminator2/1
  gbe01/2 -> Terminator1/1
  gbe01/3 -> Terminator11/1
  gbe01/6 -> Terminator5/1
  gbe01/7 -> Terminator4/1
  gbe01/8 -> Terminator90/1
  gbe01/10 -> Terminator7/1
  gbe01/11 -> Terminator8/1
  [cnt_rst] -> gbe01/1
  Constant3/1 -> gbe00/7
  ips/1(ip) -> [tx_ip], Scope3/3
  ip_counter/1 -> ips/1(ip1_sel), Scope3/2
  [cnt_rst] -> ip_counter/1, ip_counter1/1
  chSel/1(tx_valid) -> [tx_valid]  "valid1"
  [tx_ip] -> Delay3/1  "ip"
  [tx_port] -> Delay4/1  "port"
  [tx_ip] -> Delay7/1
  [tx_port2] -> Delay8/1
  chSel/2(tx_valid2) -> [tx_valid2]  "valid2"
  [tx_eof10g2] -> Delay9/1
  [tx_eof10g] -> Delay5/1  "eof"
  packetBuffer/1(dataOut) -> [tx_data1b]
  [tx_data1] -> Delay1/1  "data"
  [tx_data2] -> Delay6/1
  packetBuffer/2(dataOut1) -> [tx_data2b]
  [tx_valid] -> packetBuffer/1(enable)
  packetBuffer/3(tx_valid10g) -> [tx_valid10g]
  packetBuffer/4(tx_valid10g2) -> [tx_valid10g2]
  packetBuffer/5(tx_eof10g) -> [tx_eof10g]
  packetBuffer/6(tx_eof10g2) -> [tx_eof10g2]
  [tx_valid2] -> packetBuffer/2(enable2)
  [tx_data1a] -> packetBuffer/3(data1a)
  [tx_data2a] -> packetBuffer/4(data2a)
  [tx_data3a] -> packetBuffer/5(data3a)
  [tx_data4a] -> packetBuffer/6(data4a)
  [tx_eof10g2] -> Scope2/2, Convert5/1
  packetBuffer/7(tx_header) -> [tx_header1]
  packetBuffer/8(tx_header2) -> [tx_header2]
  [tx_header2] -> header/3(header2)
  [tx_header1] -> header/2(header1)
  [sync_rnd] -> header/1(sync_rnd)
  [tx_data1b] -> header/4(data1b)
  [tx_data2b] -> header/5(data2b)
  header/1(data1) -> [tx_data1]
  header/2(data2) -> [tx_data2]
  [tx_valid10g] -> Logical2/1  "valid"
  Logical2/1 -> gbe00/3, Scope/2, Scope4/2  "valid1"
  [tx_valid10g2] -> Logical3/1
  Logical3/1 -> gbe01/3, Scope1/2, Scope4/5  "valid2"
  header/3(validh1) -> [tx_validh1]
  header/4(validh2) -> [tx_validh2]
  [tx_validh1] -> Logical2/2
  [tx_validh2] -> Logical3/2
  Delay1/1 -> gbe00/2, Scope/1, Scope4/1  "data1"
  Delay3/1 -> gbe00/4, Scope/4  "txip"
  Delay4/1 -> gbe00/5, Scope/5  "txport"
  Delay5/1 -> gbe00/6, Scope/3, Scope4/3  "eof1"
  Delay6/1 -> Scope1/1, gbe01/2, Scope4/4  "data2"
  Delay7/1 -> gbe01/4, Scope1/4
  Delay8/1 -> gbe01/5, Scope1/5
  Delay9/1 -> gbe01/6, Scope1/3, Scope4/6  "eof2"
  [eq_out1] -> Delay10/1
  Delay10/1 -> [tx_data2a], Scope5/2
  [eq_out2] -> Delay11/1
  Delay11/1 -> [tx_data3a], Scope5/3
  [eq_out3] -> Delay12/1
  Delay12/1 -> [tx_data4a], Scope5/4
  [eq_out] -> Delay13/1
  Delay13/1 -> [tx_data1a], Scope5/1  "data1"
  Convert5/1 -> ip_counter1/2  "increment300counter"
  edge_detect3/1(out) -> ip_counter/2, Scope3/1
  ip_counter1/1 -> Relational5/1
  Relational5/1 -> edge_detect3/1(in)
  Constant1/1 -> Relational5/2
  ips/2(port) -> [tx_port], [tx_port2]

== system l64_dev/fft/sync_gen ==
  arm : Inport
  pps : Inport  Port=2
  Constant : xbsIndex_r4/Constant  const=2^sync_period_bits  gui_display_data_type=Fixed-point  arith_type=Unsigned  n_bits=sync_period_bits+1  bin_pt=0  preci_type=Single  exp_width=8  frac_width=24  explicit_period=on  period=1  equ=P=C  opselect=C  inp2=PCIN>>17  opr=+  inp1=P  carry=CIN  dbl_ovrd=off  block_type=constant
  Delay1 : xbsIndex_r4/Delay  rst=off  infoeditControl=Selection of Reset will increase slice count due to use of real FFs and instead of SRLs  en=off  latency=1  dbl_ovrd=off  reg_retiming=on  block_type=delay
  Delay2 : xbsIndex_r4/Delay  rst=off  infoeditControl=Selection of Reset will increase slice count due to use of real FFs and instead of SRLs  en=off  latency=1  dbl_ovrd=off  reg_retiming=on  block_type=delay
  rst_gen : Subsystem  mask{reset_period=1}
      mask prompts: reset_period "Min period of reset (pps pulses)"
      mask init:
      | %reset_period = eval(get_param(gcb,'reset_period'))
      | %bits = ceil(log2(reset_period))
      | %set_param([gcb,'/Counter'],'n_bits',num2str(bits));
      | %set_param([gcb,'/Counter'],'start_count', num2str(reset_period))
      | %set_param([gcb,'/Constant'],'n_bits',num2str(bits));
  sync_gen : Subsystem  mask{sync_gen_bits=sync_period_bits+1}
      mask prompts: sync_gen_bits "Size of sync generator counter"
  mrst : Outport
  sync : Outport  Port=2
  wires:
  arm/1 -> rst_gen/1(arm)
  pps/1 -> rst_gen/2(sync_in)
  sync_gen/1(sync) -> Delay2/1
  rst_gen/1(mrst) -> sync_gen/1(rst), Delay1/1
  Delay1/1 -> mrst/1
  Delay2/1 -> sync/1
  Constant/1 -> sync_gen/2(sync_period)

== system l64_dev/misc/edge_detect1 ==
  in : Inport
  Delay : xbsIndex_r4/Delay  rst=off  infoeditControl=Selection of Reset will increase slice count due to use of real FFs and instead of SRLs  en=off  latency=1  dbl_ovrd=off  reg_retiming=off  block_type=delay
      settings: xl_area=[0, 0, 0, 0, 0, 0, 0]
  Inverter : xbsIndex_r4/Inverter  en=off  latency=0  dbl_ovrd=off  block_type=inv
      settings: xl_area=[0, 0, 0, 0, 0, 0, 0]
  edge_op : xbsIndex_r4/Logical  logical_function=NOR  inputs=2  en=off  latency=0  precision=Full  arith_type=Unsigned  n_bits=8  bin_pt=2  align_bp=on  dbl_ovrd=off  block_type=logical
      settings: xl_area=[0, 0, 0, 0, 0, 0, 0]
  out : Outport
  wires:
  Inverter/1 -> edge_op/1
  edge_op/1 -> out/1
  in/1 -> Inverter/1, Delay/1
  Delay/1 -> edge_op/2

== system l64_dev/misc/edge_detect11 ==
  in : Inport
  Delay : xbsIndex_r4/Delay  rst=off  infoeditControl=Selection of Reset will increase slice count due to use of real FFs and instead of SRLs  en=off  latency=1  dbl_ovrd=off  reg_retiming=off  block_type=delay
      settings: xl_area=[0, 0, 0, 0, 0, 0, 0]
  Inverter : xbsIndex_r4/Inverter  en=off  latency=0  dbl_ovrd=off  block_type=inv
      settings: xl_area=[0, 0, 0, 0, 0, 0, 0]
  edge_op : xbsIndex_r4/Logical  logical_function=NOR  inputs=2  en=off  latency=0  precision=Full  arith_type=Unsigned  n_bits=8  bin_pt=2  align_bp=on  dbl_ovrd=off  block_type=logical
      settings: xl_area=[0, 0, 0, 0, 0, 0, 0]
  out : Outport
  wires:
  Inverter/1 -> edge_op/1
  edge_op/1 -> out/1
  in/1 -> Inverter/1, Delay/1
  Delay/1 -> edge_op/2

== system l64_dev/misc/edge_detect2 ==
  in : Inport
  Delay : xbsIndex_r4/Delay  rst=off  infoeditControl=Selection of Reset will increase slice count due to use of real FFs and instead of SRLs  en=off  latency=1  dbl_ovrd=off  reg_retiming=off  block_type=delay
      settings: xl_area=[0, 0, 0, 0, 0, 0, 0]
  Inverter : xbsIndex_r4/Inverter  en=off  latency=0  dbl_ovrd=off  block_type=inv
      settings: xl_area=[0, 0, 0, 0, 0, 0, 0]
  edge_op : xbsIndex_r4/Logical  logical_function=NOR  inputs=2  en=off  latency=0  precision=Full  arith_type=Unsigned  n_bits=8  bin_pt=2  align_bp=on  dbl_ovrd=off  block_type=logical
      settings: xl_area=[0, 0, 0, 0, 0, 0, 0]
  out : Outport
  wires:
  Inverter/1 -> edge_op/1
  edge_op/1 -> out/1
  in/1 -> Inverter/1, Delay/1
  Delay/1 -> edge_op/2

== system l64_dev/misc/edge_detect3 ==
  in : Inport
  Delay : xbsIndex_r4/Delay  rst=off  infoeditControl=Selection of Reset will increase slice count due to use of real FFs and instead of SRLs  en=off  latency=1  dbl_ovrd=off  reg_retiming=off  block_type=delay
      settings: xl_area=[0, 0, 0, 0, 0, 0, 0]
  Inverter : xbsIndex_r4/Inverter  en=off  latency=0  dbl_ovrd=off  block_type=inv
      settings: xl_area=[0, 0, 0, 0, 0, 0, 0]
  edge_op : xbsIndex_r4/Logical  logical_function=NOR  inputs=2  en=off  latency=0  precision=Full  arith_type=Unsigned  n_bits=8  bin_pt=2  align_bp=on  dbl_ovrd=off  block_type=logical
      settings: xl_area=[0, 0, 0, 0, 0, 0, 0]
  out : Outport
  wires:
  Inverter/1 -> edge_op/1
  edge_op/1 -> out/1
  in/1 -> Inverter/1, Delay/1
  Delay/1 -> edge_op/2
